simulink model "diagbloque2"  (R2019b)
settings: Solver=VariableStepAuto  StartTime=0.0  StopTime=10  RelTol=1e-3  EnableMultiTasking=on
values from neighbouring files (symbols this model uses):
  ba = 0.001    [TPpelotita.m]
  bp = 1.59    [TPpelotita.m]
  m = 0.0585    [TPpelotita.m]
  r = 0.063/2    (= 0.0315)    [TPpelotita.m]
  v0y = -100    [TPpelotita.m]
  y0 = 1.5    [TPpelotita.m]
settings Model: Creator=Paula  LastModifiedBy=Fer
settings DataIOCC: ReturnWorkspaceOutputs=off
settings OptimizationCC: LifeSpan=inf
settings DebuggingCC: SFUnexpectedBacktrackingDiag=warning  SFNoUnconditionalDefaultTransitionDiag=warning  ArithmeticOperatorsInVariantConditions=warning
settings SFSimCC: SimUseLocalCustomCode=off  CustomCodeUndefinedFunction=UseInterfaceOnly
settings RTWCC: RTWUseLocalCustomCode=off
settings CodeAppCC: StateflowObjectComments=on
settings GRTTargetCC: TargetLangStandard=C89/C90 (ANSI)  GeneratePreprocessorConditionals=Disable all
settings ConfigComp: CovMetricSettings=dw  CovHtmlReporting=on  CovSaveCumulativeToWorkspaceVar=on  CovSaveSingleToWorkspaceVar=on  CovExternalEMLEnable=off

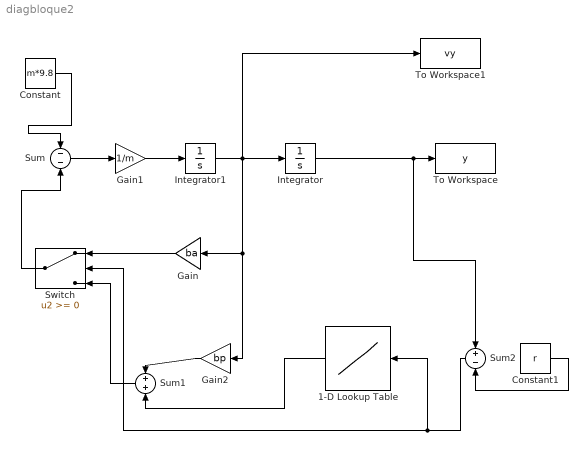
== system diagbloque2 ==
  1-D Lookup Table : Lookup_n-D  NumberOfTableDimensions=1  BreakpointsForDimension1=[0.000152979,0.000299869,0.000439218,0.000573908,0.000701165,0.000827118,0.000954278,0.001083536,0.001209584,0.001340158,0.001478477,0.00161775,0.001752221,0.001887395,0.002024889]  Table=[0.0686,0.4214,1.029,1.8424,3.0282,4.4492,6.0564,7.84,10.241,12.74,14.798,16.905,19.6392,22.344,24.843]  InternalRulePriority=Speed  RndMeth=Simplest  InputSameDT=on
  Constant : Constant  Value=m*9.8
  Constant1 : Constant  Value=r
  Gain : Gain  Gain=ba
  Gain1 : Gain  Gain=1/m
  Gain2 : Gain  Gain=bp
  Integrator : Integrator  InitialCondition=y0
  Integrator1 : Integrator  InitialCondition=v0y
  Sum : Sum  Inputs=--
  Sum1 : Sum
  Sum2 : Sum  Inputs=+-
  Switch : Switch
  To Workspace : ToWorkspace  VariableName=y  SaveFormat=Structure With Time  SampleTime=0.01
  To Workspace1 : ToWorkspace  VariableName=vy  SaveFormat=Structure With Time  SampleTime=0.01
  wires:
  Switch/1 -> Sum/2
  Gain1/1 -> Integrator1/1
  Integrator1/1 -> To Workspace1/1, Gain2/1, Gain/1, Integrator/1
  Gain/1 -> Switch/1
  Gain2/1 -> Sum1/1
  Sum1/1 -> Switch/3
  1-D Lookup Table/1 -> Sum1/2
  Constant1/1 -> Sum2/2
  Sum2/1 -> 1-D Lookup Table/1, Switch/2
  Integrator/1 -> Sum2/1, To Workspace/1
  Sum/1 -> Gain1/1
  Constant/1 -> Sum/1
